simulink model "ADXL345"  (R2021a)
settings: Solver=FixedStepDiscrete  StartTime=0.0  StopTime=Inf  FixedStep=0.02  RelTol=1e-3  EnableMultiTasking=on
undefined symbols (not defined in the file): Data
libraries: simulink x5, c280xlib x3
settings Model: SimulationMode=external  ExtModeTrigDuration=8  Creator=Syed Imtiaz Ali Shah  LastModifiedBy=Syed Imtiaz Ali Shah
settings OptimizationCC: DefaultUnderspecifiedDataType=single  EnhancedBackFolding=on  PassReuseOutputArgsAs=Individual arguments  MaxStackSize=1024  OptimizeBlockOrder=speed  DifferentSizesBufferReuse=on  OptimizationCustomize=off  DenormalBehavior=FlushToZero  EfficientTunableParamExpr=on
settings DebuggingCC: ParameterTunabilityLossMsg=error
settings HardwareCC: ProdBitPerChar=16  ProdBitPerInt=16  ProdBitPerPointer=32  ProdBitPerSizeT=32  ProdBitPerPtrDiffT=32  ProdLargestAtomicInteger=Integer  ProdLargestAtomicFloat=None  ProdWordSize=16  ProdLongLongMode=on  ProdHWDeviceType=Texas Instruments->C2000
settings SFSimCC: MATLABDynamicMemAlloc=off
settings RTWCC: SystemTargetFile=ert.tlc  HardwareBoard=TI Delfino F28379D LaunchPad  TemplateMakefile=ert_default_tmf  Toolchain=Texas Instruments Code Composer Studio (C2000)
settings CodeAppCC: ForceParamTrailComments=on  IgnoreCustomStorageClasses=off  OperatorAnnotations=on  SimulinkDataObjDesc=on  SFDataObjDesc=on  InsertBlockDesc=on
settings ERTTargetCC: CodeReplacementLibrary=TI C28x  ExtMode=on  ExtModeTransport=4  ExtModeStaticAlloc=on  ExtModeStaticAllocSize=10000  ExtModeMexFile=ext_xcp  ExtModeMexArgs=1 6 5000000  ExtModeIntrfLevel=Level2 - Open

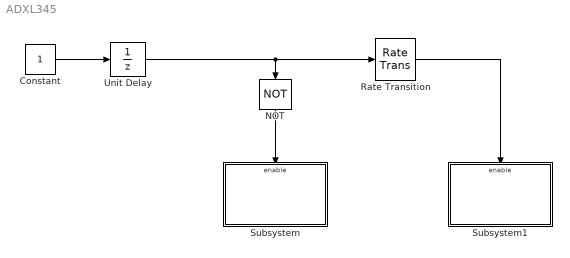
== system ADXL345 ==
  Constant : Constant
  NOT : Logic  Operator=NOT  AllPortsSameDT=off  OutDataTypeStr=boolean
  Rate Transition : RateTransition
  Subsystem : Subsystem
  Subsystem1 : Subsystem
  Unit Delay : UnitDelay  SampleTime=-1  HasFrameUpgradeWarning=on
  wires:
  Constant/1 -> Unit Delay/1
  Unit Delay/1 -> Rate Transition/1, NOT/1
  NOT/1 -> Subsystem/Enable
  Rate Transition/1 -> Subsystem1/Enable

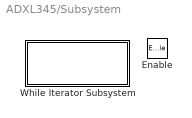
== system ADXL345/Subsystem ==
  Enable : EnablePort
  While Iterator Subsystem : Subsystem  TreatAsAtomicUnit=on

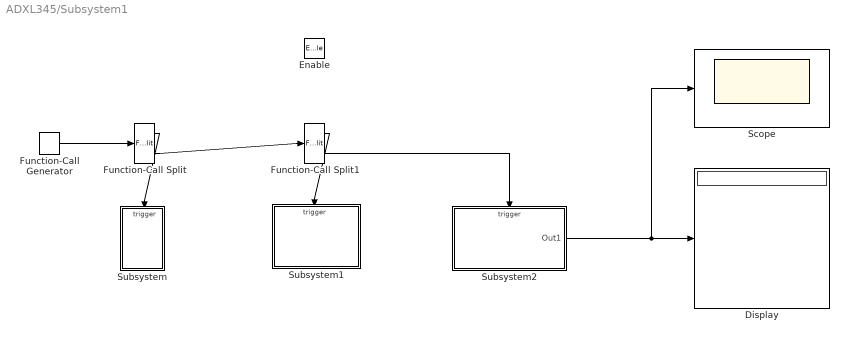
== system ADXL345/Subsystem1 ==
  Enable : EnablePort
  Display : Display
  Function-Call Generator : simulink/Ports & Subsystems/Function-Call Generator  sample_time=0.02  numberOfIterations=1  DisallowWideOutput=off
  Function-Call Split : FunctionCallSplit  NumOutputPorts=2
  Function-Call Split1 : FunctionCallSplit  NumOutputPorts=2
  Scope : Scope
  Subsystem : Subsystem
  Subsystem1 : Subsystem
  Subsystem2 : Subsystem
  wires:
  Function-Call Split/1 -> Subsystem/Trigger
  Function-Call Split1/1 -> Subsystem1/Trigger
  Function-Call Split1/2 -> Subsystem2/Trigger
  Function-Call Generator/1 -> Function-Call Split/1
  Function-Call Split/2 -> Function-Call Split1/1
  Subsystem2/1(Out1) -> Scope/1, Display/1

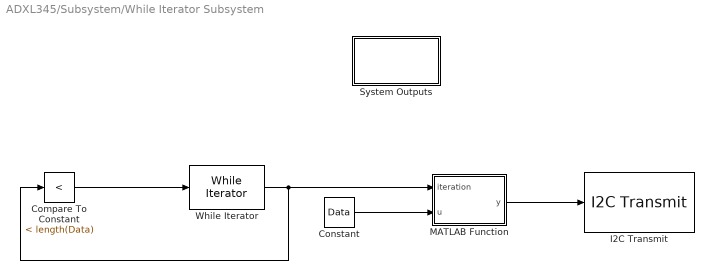
== system ADXL345/Subsystem/While Iterator Subsystem ==
  Compare To Constant : simulink/Logic and Bit Operations/Compare To Constant  relop=<  const=length(Data)  OutDataTypeStr=boolean
  Constant : Constant  Value=Data  OutDataTypeStr=uint8
  I2C Transmit : c280xlib/I2C Transmit  selectModule=I2C_A  addrFormat=7-Bit addressing  saSource=Specify via dialog  SAR=83  bitCount=8  STP=on  RM=off  STR=off
      settings: SourceProductBaseCode=TIC2000
  MATLAB Function : MATLAB Function  TreatAsAtomicUnit=on
  System Outputs : Subsystem  mask(System Outputs){ShowInLibBrowser=0}
      mask prompts: ShowInLibBrowser "Simulink:masks:CustCodeMaskParam1_MP"
      settings: CopyFcn=cccopyfcn(gcb)  OpenFcn=ccopenfcn('System Outputs Function')
      mask Help: eval('feval(''rtwprivate'',''rtwhelpview'',''rtw_sys_outputs_block'')');
      mask Display: disp('System\nOutputs');
  While Iterator : WhileIterator  MaxIters=-1  WhileBlockType=do-while  ShowIterationPort=on
  wires:
  MATLAB Function/1(y) -> I2C Transmit/1
  Constant/1 -> MATLAB Function/2(u)
  Compare To Constant/1 -> While Iterator/1
  While Iterator/1 -> MATLAB Function/1(iteration), Compare To Constant/1

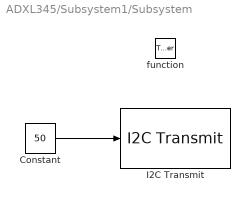
== system ADXL345/Subsystem1/Subsystem ==
  function : TriggerPort  TriggerType=function-call  VariantControl=(inherit)
  Constant : Constant  Value=50  OutDataTypeStr=uint8
  I2C Transmit : c280xlib/I2C Transmit  selectModule=I2C_A  addrFormat=7-Bit addressing  saSource=Specify via dialog  SAR=83  bitCount=8  STP=off  RM=off  STR=off
      settings: SourceProductBaseCode=TIC2000
  wires:
  Constant/1 -> I2C Transmit/1

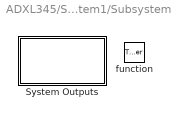
== system ADXL345/Subsystem1/Subsystem1 ==
  function : TriggerPort  TriggerType=function-call  VariantControl=(inherit)
  System Outputs : Subsystem  mask(System Outputs){ShowInLibBrowser=0}
      mask prompts: ShowInLibBrowser "Simulink:masks:CustCodeMaskParam1_MP"
      settings: CopyFcn=cccopyfcn(gcb)  OpenFcn=ccopenfcn('System Outputs Function')
      mask Help: eval('feval(''rtwprivate'',''rtwhelpview'',''rtw_sys_outputs_block'')');
      mask Display: disp('System\nOutputs');

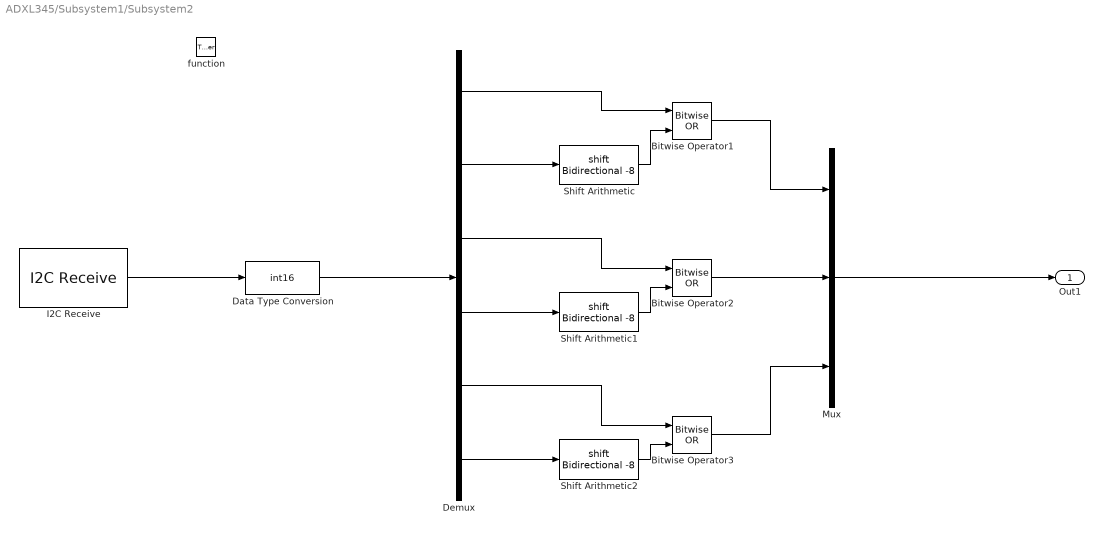
== system ADXL345/Subsystem1/Subsystem2 ==
  function : TriggerPort  TriggerType=function-call  VariantControl=(inherit)
  Bitwise Operator1 : simulink/Logic and Bit Operations/Bitwise Operator  logicop=OR  UseBitMask=off  NumInputPorts=2  BitMask=bin2dec('11011001')  BitMaskRealWorld=Stored Integer
  Bitwise Operator2 : simulink/Logic and Bit Operations/Bitwise Operator  logicop=OR  UseBitMask=off  NumInputPorts=2  BitMask=bin2dec('11011001')  BitMaskRealWorld=Stored Integer
  Bitwise Operator3 : simulink/Logic and Bit Operations/Bitwise Operator  logicop=OR  UseBitMask=off  NumInputPorts=2  BitMask=bin2dec('11011001')  BitMaskRealWorld=Stored Integer
  Data Type Conversion : DataTypeConversion  OutDataTypeStr=int16  ConvertRealWorld=Stored Integer (SI)
  Demux : Demux  Outputs=6
  I2C Receive : c280xlib/I2C Receive  selectModule=I2C_A  addrFormat=7-Bit addressing  saSource=Specify via dialog  SAR=83  bitCount=8  dataLength=6  initValue=0  NACK=off  STP=on  STR=off  sampleTime=-1  dataType=uint8
      settings: SourceProductBaseCode=TIC2000
  Mux : Mux  Inputs=3
  Shift Arithmetic : ArithShift  BitShiftNumber=-8
  Shift Arithmetic1 : ArithShift  BitShiftNumber=-8
  Shift Arithmetic2 : ArithShift  BitShiftNumber=-8
  Out1 : Outport
  wires:
  I2C Receive/1 -> Data Type Conversion/1
  Shift Arithmetic2/1 -> Bitwise Operator3/2
  Demux/4 -> Shift Arithmetic1/1
  Bitwise Operator3/1 -> Mux/3
  Shift Arithmetic/1 -> Bitwise Operator1/2
  Shift Arithmetic1/1 -> Bitwise Operator2/2
  Demux/6 -> Shift Arithmetic2/1
  Demux/3 -> Bitwise Operator2/1
  Bitwise Operator2/1 -> Mux/2
  Demux/5 -> Bitwise Operator3/1
  Data Type Conversion/1 -> Demux/1
  Demux/1 -> Bitwise Operator1/1
  Demux/2 -> Shift Arithmetic/1
  Bitwise Operator1/1 -> Mux/1
  Mux/1 -> Out1/1

== system ADXL345/Subsystem/While Iterator Subsystem/System Outputs ==

== system ADXL345/Subsystem1/Subsystem1/System Outputs ==

== matlab function ADXL345/Subsystem/While Iterator Subsystem/MATLAB Function ==
  data: iteration input; u input; y output
function y = fcn(iteration, u)
y = [u((iteration),1) u((iteration),2)];
